simulink model "steamjacket"  (R2021b)
settings: Solver=VariableStepAuto  StartTime=0.0  StopTime=10.0  RelTol=1e-3
settings Model: Creator=Edwar  LastModifiedBy=Edwar

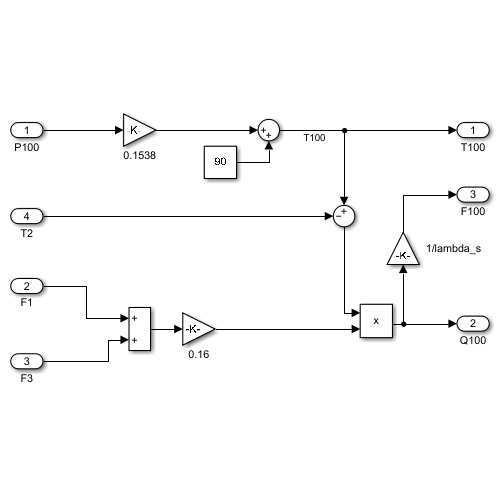
[thumbnail: Simulink's stored preview of the top-level diagram]
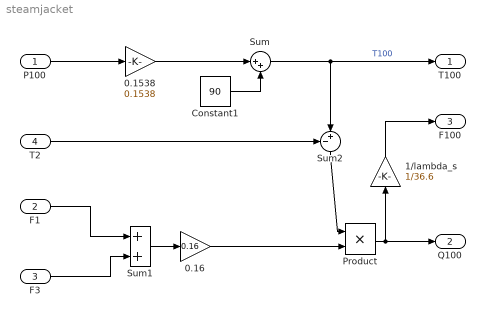
== system steamjacket ==
  P100 : Inport
  F1 : Inport  Port=2
  F3 : Inport  Port=3
  T2 : Inport  Port=4
  0.1538 : Gain  Gain=0.1538
  0.16 : Gain  Gain=0.16
  1/lambda_s : Gain  Gain=1/36.6
  Constant1 : Constant  Value=90
  Product : Product
  Sum : Sum  Inputs=|++
  Sum1 : Sum
  Sum2 : Sum  Inputs=-+|
  T100 : Outport
  Q100 : Outport  Port=2
  F100 : Outport  Port=3
  wires:
  P100/1 -> 0.1538/1
  0.1538/1 -> Sum/1
  Constant1/1 -> Sum/2
  Sum/1 -> Sum2/2, T100/1  "T100"
  F1/1 -> Sum1/1
  F3/1 -> Sum1/2
  Sum1/1 -> 0.16/1
  T2/1 -> Sum2/1
  Sum2/1 -> Product/1
  0.16/1 -> Product/2
  Product/1 -> Q100/1, 1/lambda_s/1
  1/lambda_s/1 -> F100/1
